simulink model "PLL_tipo2"  (Simulink 7.3)
settings: Solver=ode23t  StartTime=0.0  StopTime=2  RelTol=1e-5
values from neighbouring files (symbols this model uses):
  Ts = 50e-6    (= 5e-05)    [parametros_PLL_a.m]
settings Model: Creator=nicolas  LastModifiedBy=Wassinger

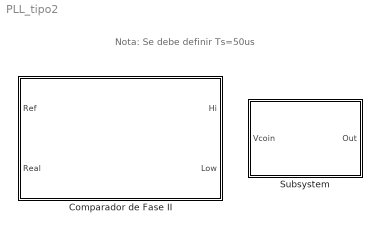
== system PLL_tipo2 ==
  note: Nota: Se debe definir Ts=50us
  Comparador de Fase II : Subsystem  mask{Ts=Ts}
      mask Display:
      | disp('Comparador de Fase II')
      | port_label('input',1,'Referencia')
      | port_label('input',2,'Relimentación')
      | port_label('output',1,'Hi_Switch')
      | port_label('output',2,'Low_Switch')
  Subsystem : Subsystem  mask{Ts=Ts}
      mask Display:
      | disp('VCO')
      | port_label('input',1,'Vcoin')
      | port_label('output',1,'Out')

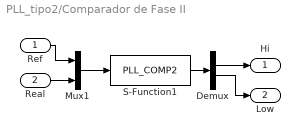
== system PLL_tipo2/Comparador de Fase II ==
  Ref : Inport
  Real : Inport  Port=2
  Demux : Demux
  Mux1 : Mux  Inputs=2
  S-Function1 : S-Function  FunctionName=PLL_COMP2  Parameters=Ts  EnableBusSupport=off
  Hi : Outport
  Low : Outport  Port=2
  wires:
  Mux1/1 -> S-Function1/1
  S-Function1/1 -> Demux/1
  Ref/1 -> Mux1/1
  Demux/2 -> Hi/1
  Demux/3 -> Low/1
  Real/1 -> Mux1/2

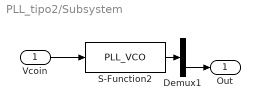
== system PLL_tipo2/Subsystem ==
  Vcoin : Inport
  Demux1 : Demux  Outputs=2
  S-Function2 : S-Function  FunctionName=PLL_VCO  Parameters=Ts  EnableBusSupport=off
  Out : Outport
  wires:
  S-Function2/1 -> Demux1/1
  Vcoin/1 -> S-Function2/1
  Demux1/2 -> Out/1
